simulink model "Roadsense_ClosedLoopIntegration"  (R2025b)
settings: Solver=FixedStepDiscrete  StartTime=0.0  StopTime=2.0  FixedStep=RsTsBase  RelTol=1e-3
undefined symbols (not defined in the file or in its folder): RsTsBase, RsTsControl, RsTsFusion
settings Model: DataDictionary=Roadsense_Data.sldd  Creator=ragur  LastModifiedBy=ragur

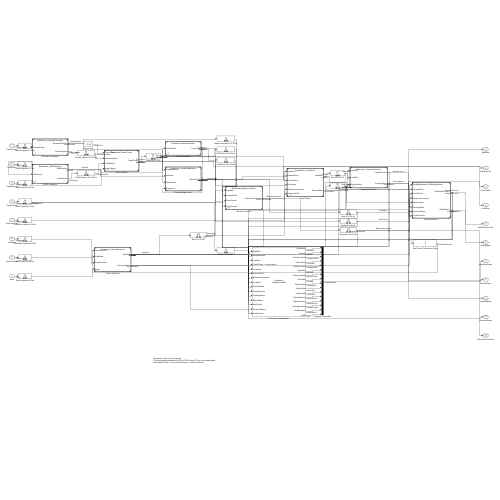
[thumbnail: Simulink's stored preview of the top-level diagram]
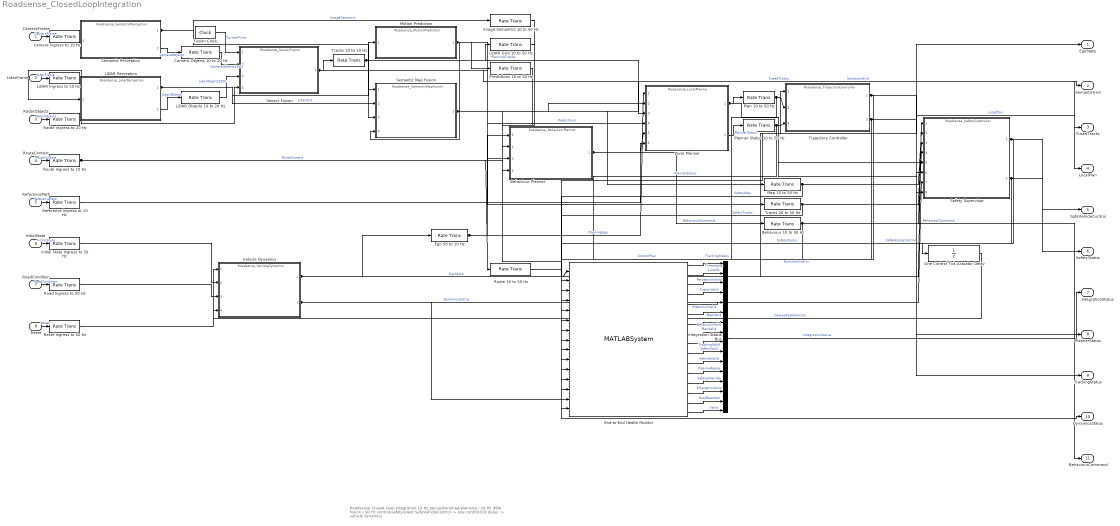
== system Roadsense_ClosedLoopIntegration ==
  note: Roadsense Closed-Loop Integration
      | 10 Hz perception/map/planning | 20 Hz JPDA fusion | 50 Hz control/safety/plant
      | SafeVehicleControl -> one control-tick delay -> vehicle dynamics
  CameraFrame : Inport  OutDataTypeStr=Bus: RsCameraFrameBus  PortDimensions=1  SampleTime=RsTsBase
  LidarFrame : Inport  Port=2  OutDataTypeStr=Bus: RsLidarFrameBus  PortDimensions=1  SampleTime=RsTsBase
  RadarObjects : Inport  Port=3  OutDataTypeStr=Bus: RsRadarObjectListBus  PortDimensions=1  SampleTime=RsTsBase
  RouteContext : Inport  Port=4  OutDataTypeStr=Bus: RsRouteContextBus  PortDimensions=1  SampleTime=RsTsBase
  ReferencePath : Inport  Port=5  OutDataTypeStr=Bus: RsReferencePathBus  PortDimensions=1  SampleTime=RsTsBase
  InitialState : Inport  Port=6  OutDataTypeStr=Bus: RsEgoStateBus  PortDimensions=1  SampleTime=RsTsBase
  RoadCondition : Inport  Port=7  OutDataTypeStr=Bus: RsRoadConditionBus  PortDimensions=1  SampleTime=RsTsBase
  Reset : Inport  Port=8  OutDataTypeStr=boolean  PortDimensions=1  SampleTime=RsTsBase
  Behaviour 10 to 50 Hz : RateTransition  OutPortSampleTime=RsTsControl
  Behaviour Planner : ModelReference  ModelNameDialog=Roadsense_BehaviourPlanner  SimulationMode=Normal  ModelReferenceVersion=1.1
  Camera Ingress to 10 Hz : RateTransition  OutPortSampleTime=RsTsSemanticInference
  Camera Objects 10 to 20 Hz : RateTransition  OutPortSampleTime=RsTsFusion
  Ego 50 to 10 Hz : RateTransition  OutPortSampleTime=RsTsPlanning
  End-to-End Health Monitor : MATLABSystem  System=RoadsenseIntegrationMonitorSystem  SimulateUsing=Code generation
      mask Type: RoadsenseIntegrationMonitorSystem
  Fusion Clock : DigitalClock  SampleTime=RsTsFusion
  Image Semantics 10 to 50 Hz : RateTransition  OutPortSampleTime=RsTsControl
  Initial State Ingress to 50 Hz : RateTransition  OutPortSampleTime=RsTsControl
  Integration Status Bus : BusCreator  Inputs=16  OutDataTypeStr=Bus: RsIntegrationStatusBus
  LiDAR Grid 10 to 50 Hz : RateTransition  OutPortSampleTime=RsTsControl
  LiDAR Ingress to 10 Hz : RateTransition  OutPortSampleTime=RsTsLidarPerception
  LiDAR Objects 10 to 20 Hz : RateTransition  OutPortSampleTime=RsTsFusion
  LiDAR Perception : ModelReference  ModelNameDialog=Roadsense_LidarPerception  SimulationMode=Normal  ModelReferenceVersion=1.1
  Local Planner : ModelReference  ModelNameDialog=Roadsense_LocalPlanner  SimulationMode=Normal  ModelReferenceVersion=1.1
  Map 10 to 50 Hz : RateTransition  OutPortSampleTime=RsTsControl
  Motion Prediction : ModelReference  ModelNameDialog=Roadsense_MotionPrediction  SimulationMode=Normal  ModelReferenceVersion=1.1
  One Control Tick Actuator Delay : UnitDelay  SampleTime=RsTsControl  HasFrameUpgradeWarning=on
  Plan 10 to 50 Hz : RateTransition  OutPortSampleTime=RsTsControl
  Planner Status 10 to 50 Hz : RateTransition  OutPortSampleTime=RsTsControl
  Predictions 10 to 50 Hz : RateTransition  OutPortSampleTime=RsTsControl
  Radar Ingress to 20 Hz : RateTransition  OutPortSampleTime=RsTsFusion
  Reference Ingress to 10 Hz : RateTransition  OutPortSampleTime=RsTsPlanning
  Reset Ingress to 50 Hz : RateTransition  OutPortSampleTime=RsTsControl
  Road Ingress to 50 Hz : RateTransition  OutPortSampleTime=RsTsControl
  Route 10 to 50 Hz : RateTransition  OutPortSampleTime=RsTsControl
  Route Ingress to 10 Hz : RateTransition  OutPortSampleTime=RsTsPlanning
  Safety Supervisor : ModelReference  ModelNameDialog=Roadsense_SafetySupervisor  SimulationMode=Normal  ModelReferenceVersion=1.1
  Semantic Map Fusion : ModelReference  ModelNameDialog=Roadsense_SemanticMapFusion  SimulationMode=Normal  ModelReferenceVersion=1.1
  Semantic Perception : ModelReference  ModelNameDialog=Roadsense_SemanticPerception  SimulationMode=Normal  ModelReferenceVersion=1.1
  Sensor Fusion : ModelReference  ModelNameDialog=Roadsense_SensorFusion  SimulationMode=Normal  ModelReferenceVersion=1.1
  Tracks 20 to 10 Hz : RateTransition  OutPortSampleTime=RsTsPlanning
  Tracks 20 to 50 Hz : RateTransition  Deterministic=off  OutPortSampleTime=RsTsControl
  Trajectory Controller : ModelReference  ModelNameDialog=Roadsense_TrajectoryController  SimulationMode=Normal  ModelReferenceVersion=1.1
  Vehicle Dynamics : ModelReference  ModelNameDialog=Roadsense_VehicleDynamics  SimulationMode=Normal  ModelReferenceVersion=1.1
  EgoState : Outport  OutDataTypeStr=Bus: RsEgoStateBus
  SemanticGrid : Outport  Port=2  OutDataTypeStr=Bus: RsSemanticGridBus
  FusedTracks : Outport  Port=3  OutDataTypeStr=Bus: RsFusedTrackListBus
  LocalPlan : Outport  Port=4  OutDataTypeStr=Bus: RsLocalPlanBus
  SafeVehicleControl : Outport  Port=5  OutDataTypeStr=Bus: RsVehicleControlBus
  SafetyStatus : Outport  Port=6  OutDataTypeStr=Bus: RsSafetyStatusBus
  IntegrationStatus : Outport  Port=7  OutDataTypeStr=Bus: RsIntegrationStatusBus
  PlannerStatus : Outport  Port=8  OutDataTypeStr=Bus: RsPlannerStatusBus
  TrackingStatus : Outport  Port=9  OutDataTypeStr=Bus: RsTrackingStatusBus
  DynamicsStatus : Outport  Port=10  OutDataTypeStr=Bus: RsVehicleDynamicsStatusBus
  BehaviourCommand : Outport  Port=11  OutDataTypeStr=Bus: RsBehaviourCommandBus
  wires:
  CameraFrame/1 -> Camera Ingress to 10 Hz/1  "CameraFrame"
  Camera Ingress to 10 Hz/1 -> Semantic Perception/1
  LidarFrame/1 -> LiDAR Ingress to 10 Hz/1  "LidarFrame"
  LiDAR Ingress to 10 Hz/1 -> LiDAR Perception/1
  Semantic Perception/2 -> Camera Objects 10 to 20 Hz/1  "CameraObjects"
  Fusion Clock/1 -> Sensor Fusion/1  "CurrentTime"
  Camera Objects 10 to 20 Hz/1 -> Sensor Fusion/2  "CameraObjects20Hz"
  LiDAR Perception/2 -> LiDAR Objects 10 to 20 Hz/1  "LidarObjects"
  LiDAR Objects 10 to 20 Hz/1 -> Sensor Fusion/3  "LidarObjects20Hz"
  RadarObjects/1 -> Radar Ingress to 20 Hz/1  "RadarObjects"
  Radar Ingress to 20 Hz/1 -> Sensor Fusion/4
  Sensor Fusion/1 -> Tracks 20 to 10 Hz/1, Tracks 20 to 50 Hz/1, FusedTracks/1  "FusedTracks"
  Tracks 20 to 10 Hz/1 -> Motion Prediction/1, Semantic Map Fusion/3, Behaviour Planner/3, Local Planner/3  "PlanningTracks"
  Semantic Perception/1 -> Semantic Map Fusion/1, Image Semantics 10 to 50 Hz/1  "ImageSemantic"
  LiDAR Perception/1 -> Semantic Map Fusion/2, LiDAR Grid 10 to 50 Hz/1  "LidarGrid"
  Motion Prediction/1 -> Semantic Map Fusion/4, Local Planner/4, Predictions 10 to 50 Hz/1  "Predictions"
  Vehicle Dynamics/1 -> Ego 50 to 10 Hz/1, Trajectory Controller/1, Safety Supervisor/1, End-to-End Health Monitor/1, EgoState/1  "EgoState"
  Ego 50 to 10 Hz/1 -> Behaviour Planner/1, Local Planner/1  "PlanningEgo"
  Semantic Map Fusion/1 -> Behaviour Planner/2, Local Planner/2, Map 10 to 50 Hz/1, SemanticGrid/1  "SemanticGrid"
  RouteContext/1 -> Route Ingress to 10 Hz/1  "RouteContext"
  Route Ingress to 10 Hz/1 -> Behaviour Planner/4, Route 10 to 50 Hz/1  "RouteContext"
  Behaviour Planner/1 -> Local Planner/5, Behaviour 10 to 50 Hz/1  "BehaviourCommand"
  ReferencePath/1 -> Reference Ingress to 10 Hz/1  "ReferencePath"
  Reference Ingress to 10 Hz/1 -> Local Planner/6
  Local Planner/1 -> Plan 10 to 50 Hz/1, LocalPlan/1  "LocalPlan"
  Local Planner/2 -> Planner Status 10 to 50 Hz/1  "PlannerStatus"
  Plan 10 to 50 Hz/1 -> Trajectory Controller/2, End-to-End Health Monitor/8  "ControlPlan"
  Planner Status 10 to 50 Hz/1 -> Trajectory Controller/3, Safety Supervisor/5, End-to-End Health Monitor/9, PlannerStatus/1  "PlannerStatus"
  Map 10 to 50 Hz/1 -> Safety Supervisor/2, End-to-End Health Monitor/6  "SafetyMap"
  Tracks 20 to 50 Hz/1 -> Safety Supervisor/3, End-to-End Health Monitor/4  "SafetyTracks"
  Behaviour 10 to 50 Hz/1 -> Safety Supervisor/4, End-to-End Health Monitor/7, BehaviourCommand/1  "BehaviourCommand"
  Trajectory Controller/2 -> Safety Supervisor/6, End-to-End Health Monitor/11, TrackingStatus/1  "TrackingStatus"
  Vehicle Dynamics/2 -> Safety Supervisor/7, End-to-End Health Monitor/14, DynamicsStatus/1  "DynamicsStatus"
  Trajectory Controller/1 -> Safety Supervisor/8, End-to-End Health Monitor/10  "NominalControl"
  Safety Supervisor/1 -> One Control Tick Actuator Delay/1, End-to-End Health Monitor/13, SafeVehicleControl/1  "SafeVehicleControl"
  One Control Tick Actuator Delay/1 -> Vehicle Dynamics/1  "DelayedSafeControl"
  InitialState/1 -> Initial State Ingress to 50 Hz/1  "InitialState"
  Initial State Ingress to 50 Hz/1 -> Vehicle Dynamics/2
  RoadCondition/1 -> Road Ingress to 50 Hz/1  "RoadCondition"
  Road Ingress to 50 Hz/1 -> Vehicle Dynamics/3
  Reset/1 -> Reset Ingress to 50 Hz/1  "Reset"
  Reset Ingress to 50 Hz/1 -> Vehicle Dynamics/4
  Image Semantics 10 to 50 Hz/1 -> End-to-End Health Monitor/2
  LiDAR Grid 10 to 50 Hz/1 -> End-to-End Health Monitor/3
  Predictions 10 to 50 Hz/1 -> End-to-End Health Monitor/5
  Safety Supervisor/2 -> End-to-End Health Monitor/12, SafetyStatus/1  "SafetyStatus"
  Route 10 to 50 Hz/1 -> End-to-End Health Monitor/15
  End-to-End Health Monitor/1 -> Integration Status Bus/1  "Timestamp"
  End-to-End Health Monitor/2 -> Integration Status Bus/2  "CycleID"
  End-to-End Health Monitor/3 -> Integration Status Bus/3  "PerceptionValid"
  End-to-End Health Monitor/4 -> Integration Status Bus/4  "FusionValid"
  End-to-End Health Monitor/5 -> Integration Status Bus/5  "PredictionValid"
  End-to-End Health Monitor/6 -> Integration Status Bus/6  "MapValid"
  End-to-End Health Monitor/7 -> Integration Status Bus/7  "BehaviourValid"
  End-to-End Health Monitor/8 -> Integration Status Bus/8  "PlanValid"
  End-to-End Health Monitor/9 -> Integration Status Bus/9  "TrackingValid"
  End-to-End Health Monitor/10 -> Integration Status Bus/10  "SafetyValid"
  End-to-End Health Monitor/11 -> Integration Status Bus/11  "VehicleValid"
  End-to-End Health Monitor/12 -> Integration Status Bus/12  "PipelineReady"
  End-to-End Health Monitor/13 -> Integration Status Bus/13  "SafetyOverride"
  End-to-End Health Monitor/14 -> Integration Status Bus/14  "EmergencyStop"
  End-to-End Health Monitor/15 -> Integration Status Bus/15  "GoalReached"
  End-to-End Health Monitor/16 -> Integration Status Bus/16  "Valid"
  Integration Status Bus/1 -> IntegrationStatus/1  "IntegrationStatus"
